simulink model "SimulationOfFurutaL3"  (R2017a)
settings: Solver=FixedStepAuto  StartTime=0.0  StopTime=10.0  FixedStep=0.001  RelTol=1e-3
values from neighbouring files (symbols this model uses):
  b10 = 6.05e-3    (= 0.00605)    [FurutaConstants.m]
  b20 = 5.52e-04    (= 0.000552)    [FurutaConstants.m]
  g0 = 9.81    [FurutaConstants.m]
  I2y0 = 0.2937e-3    (= 0.0002937)    [FurutaConstants.m]
  I2z0 = 0.0051e-3    (= 5.1e-06)    [FurutaConstants.m]
  Ixz20 = -0.0131e-3    (= -1.31e-05)    [FurutaConstants.m]
  k10 = (I2y0 + I1z0 + L10^2*m20+l10^2*m10+l20^2*m20)/2    (= 0.00399493504648)    [FurutaConstants.m]
  k20 = (I2x0+l20^2*m20)/2    (= 0.000230092732776)    [FurutaConstants.m]
  kt0 = 0.122326    [FurutaConstants.m]
  L10 = 230.45e-3    (= 0.23045)    [FurutaConstants.m]
  l20 = 58.18e-3    (= 0.05818)    [FurutaConstants.m]
  m20 = 0.04948    [FurutaConstants.m]
  Rm0 = 12.38    [FurutaConstants.m]
settings Model: Creator=felip  LastModifiedBy=felip

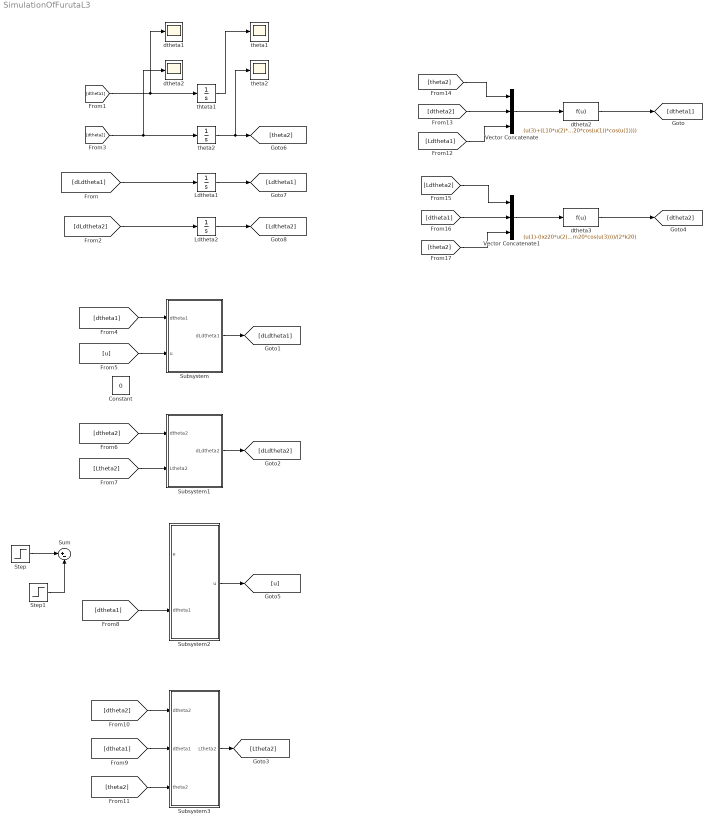
== system SimulationOfFurutaL3 ==
  Constant : Constant  Value=0
  Ldtheta1 : Integrator
  Ldtheta2 : Integrator
  Step : Step  Time=0  After=12  SampleTime=0
  Step1 : Step  Time=1/12  After=12  SampleTime=0
  Subsystem : Subsystem
  Subsystem1 : Subsystem
  Subsystem2 : Subsystem
  Subsystem3 : Subsystem
  Sum : Sum  Inputs=|+-
  Vector Concatenate : Concatenate  NumInputs=3
  Vector Concatenate1 : Concatenate  NumInputs=3
  dtheta1 : Scope
  dtheta2 : Fcn  Expr=(u(3)+(L10*u(2)*l20*m20*cos(u(1)))-(Ixz20*u(2)*cos(u(1))))/((2*k10)-(I2y0*(cos(u(1)))^2)+(I2z0*(cos(u(1)))^2)-(l20*l20*m20*cos(u(1))*cos(u(1))))
  "dtheta2 " : Scope
  dtheta3 : Fcn  Expr=(u(1)-(Ixz20*u(2)*cos(u(3)))+(L10*u(2)*l20*m20*cos(u(3))))/(2*k20)
  theta1 : Scope
  theta2 : Integrator  InitialCondition=pi
  "theta2 " : Scope
  thteta1 : Integrator
  wires:
  Ldtheta1/1 -> [Ldtheta1]
  thteta1/1 -> theta1/1
  Ldtheta2/1 -> [Ldtheta2]
  [dtheta1] -> thteta1/1, dtheta1/1
  [dLdtheta1] -> Ldtheta1/1
  theta2/1 -> [theta2], "theta2 "/1
  [dtheta2] -> "dtheta2 "/1, theta2/1
  [dLdtheta2] -> Ldtheta2/1
  [dtheta1] -> Subsystem/1(dtheta1)
  Subsystem/1(dLdtheta1) -> [dLdtheta1]
  [dtheta2] -> Subsystem1/1(dtheta2)
  [Ltheta2] -> Subsystem1/2(Ltheta2)
  Subsystem1/1(dLdtheta2) -> [dLdtheta2]
  Subsystem2/1("u ") -> [u]
  Step1/1 -> Sum/2
  Step/1 -> Sum/1
  [dtheta1] -> Subsystem2/2(dtheta1)
  Subsystem3/1("Ltheta2 ") -> [Ltheta2]
  [dtheta1] -> Subsystem3/2(dtheta1)
  [dtheta2] -> Subsystem3/1(dtheta2)
  [theta2] -> Subsystem3/3(theta2)
  [dtheta2] -> Vector Concatenate/2
  [Ldtheta1] -> Vector Concatenate/3
  [theta2] -> Vector Concatenate/1
  [dtheta1] -> Vector Concatenate1/2
  [theta2] -> Vector Concatenate1/3
  Vector Concatenate/1 -> dtheta2/1
  [Ldtheta2] -> Vector Concatenate1/1
  dtheta2/1 -> [dtheta1]
  Vector Concatenate1/1 -> dtheta3/1
  dtheta3/1 -> [dtheta2]
  [u] -> Subsystem/2(u)

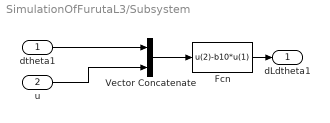
== system SimulationOfFurutaL3/Subsystem ==
  dtheta1 : Inport
  u : Inport  Port=2
  Fcn : Fcn  Expr=u(2)-b10*u(1)
  Vector Concatenate : Concatenate
  dLdtheta1 : Outport
  wires:
  Fcn/1 -> dLdtheta1/1
  dtheta1/1 -> Vector Concatenate/1
  Vector Concatenate/1 -> Fcn/1
  u/1 -> Vector Concatenate/2

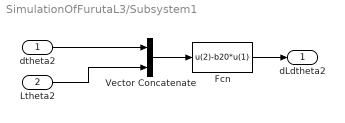
== system SimulationOfFurutaL3/Subsystem1 ==
  dtheta2 : Inport
  Ltheta2 : Inport  Port=2
  Fcn : Fcn  Expr=u(2)-b20*u(1)
  Vector Concatenate : Concatenate
  dLdtheta2 : Outport
  wires:
  Fcn/1 -> dLdtheta2/1
  dtheta2/1 -> Vector Concatenate/1
  Vector Concatenate/1 -> Fcn/1
  Ltheta2/1 -> Vector Concatenate/2

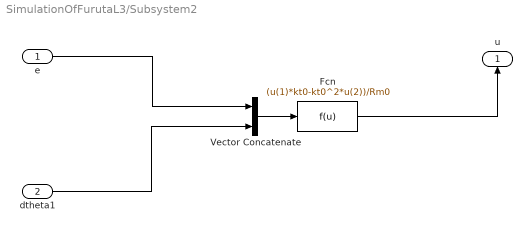
== system SimulationOfFurutaL3/Subsystem2 ==
  e : Inport
  dtheta1 : Inport  Port=2
  Fcn : Fcn  Expr=(u(1)*kt0-kt0^2*u(2))/Rm0
  Vector Concatenate : Concatenate
  "u " : Outport
  wires:
  Fcn/1 -> "u "/1
  dtheta1/1 -> Vector Concatenate/2
  Vector Concatenate/1 -> Fcn/1
  e/1 -> Vector Concatenate/1

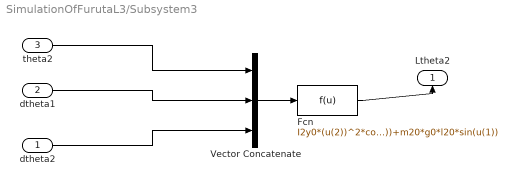
== system SimulationOfFurutaL3/Subsystem3 ==
  dtheta2 : Inport
  dtheta1 : Inport  Port=2
  theta2 : Inport  Port=3
  Fcn : Fcn  Expr=I2y0*(u(2))^2*cos(u(1))*sin(u(1))-I2z0*(u(2))^2*cos(u(1))*sin(u(1))-Ixz20*u(2)*u(3)*sin(u(1))+(u(2))^2*l20^2*m20*cos(u(1))*sin(u(1))+L10*u(2)*u(3)*l20*m20*sin(u(1))+m20*g0*l20*sin(u(1))
  Vector Concatenate : Concatenate  NumInputs=3
  "Ltheta2 " : Outport
  wires:
  Fcn/1 -> "Ltheta2 "/1
  Vector Concatenate/1 -> Fcn/1
  dtheta2/1 -> Vector Concatenate/3
  dtheta1/1 -> Vector Concatenate/2
  theta2/1 -> Vector Concatenate/1
